simulink model "UScityblock2_Intersection"  (R2021b)
settings: Solver=ode23s  StartTime=0.0  StopTime=25  RelTol=1e-3
model workspace (MAT data in the model file):
  firstWarning = 1
  originalScenarioChecksum = '44EB4239245A86A3DA7E3FEB76A9F5A7'
values from neighbouring files (symbols this model uses):
  curvature = (DX.*D2Y - DY.*D2X) ./(DX.^2+DY.^2).^(3/2)    [setUpModel_UScityblock2.m]
  direction = ones(length(gradbp),1)    [setUpModel_UScityblock2.m]
  gradbp = linspace(0,totalDistance,50)    [setUpModel_UScityblock2.m]
  psi_o = thetaRefab(1)*(pi/180)    [setUpModel_UScityblock2.m]
  speed_actor1_gdps = smooth(speedgradbpactor1,speedactor1le)    [velocity_profiles.m]
  speed_actor2_gdps = smooth(speedgradbpactor2,speedactor2le)    [velocity_profiles.m]
  speed_actor3_gdps = smooth(speedgradbpactor3,speedactor3le)    [velocity_profiles.m]
  speed_actor4_gdps = smooth(speedgradbpactor4,speedactor4le)    [velocity_profiles.m]
  speed_ego_gdps = smooth(speedgradbpego,speedegole)    [velocity_profiles.m]
  thetaRefab = zeros(length(gradbp),1)    [setUpModel_UScityblock2.m]
  x_gdps = smooth(gradbp,xwaypoints)    [setUpModel_UScityblock2.m]
  X_o = x_ego_i(1)    [setUpModel_UScityblock2.m]
  y_gdps = smooth(gradbp,ywaypoints)    [setUpModel_UScityblock2.m]
  Y_o = y_ego_i(1)    [setUpModel_UScityblock2.m]
undefined symbols (not defined in the file or in its folder): distancecovered, gradbpA1, gradbpA2, gradbpA3, gradbpA4, gradbpego, magnitude, n, q11, v2xCA
libraries: drivingscenarioandsensors x7, sim3dautolib x5, vehdynlibtirecommon x4, autolibutils x4, aerolibconvert2 x2, simulink_extras x2, drivingvehiclecontroller x2, sim3dlib x1, vehdynlibtire x1, simulink x1, autolibshared x1
(part 2 of 2)

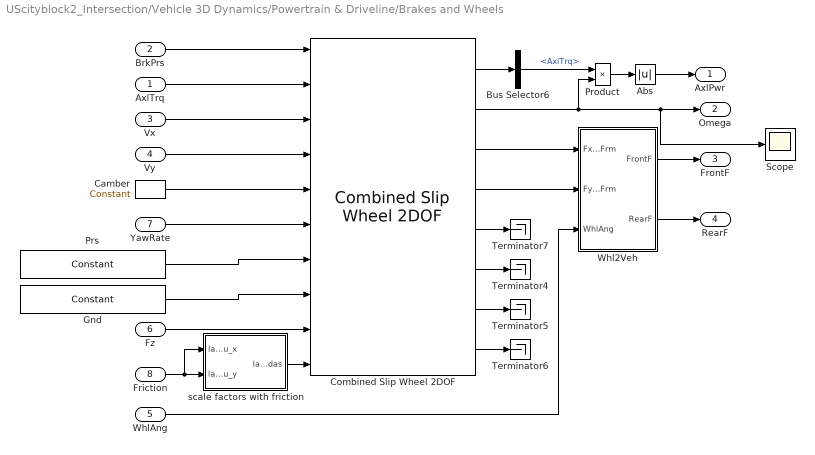
== system UScityblock2_Intersection/Vehicle 3D Dynamics/Powertrain & Driveline/Brakes and Wheels ==
  AxlTrq : Inport
  BrkPrs : Inport  Port=2
  Vx : Inport  Port=3
  Vy : Inport  Port=4
  WhlAng : Inport  Port=5
  Fz : Inport  Port=6  PortDimensions=4
  YawRate : Inport  Port=7
  Friction : Inport  Port=8
  Abs : Abs
  Bus Selector6 : BusSelector  OutputSignals=AxlTrq
  Camber : vehdynlibtirecommon/Constant  const=0  numWheels=4
      settings: SourceProductBaseCode=VE
  Combined Slip Wheel 2DOF : vehdynlibtire/Combined Slip Wheel 2DOF  tireType=External file  BrakeType=Disc  plySteer=off  turnslip=off  mu_static=.3  mu_kinetic=.2  disk_abore=.05  Rm=.177  num_pads=2  drum_abore=0.0508  drum_a=0.123  drum_c=0.212  drum_r=0.15  drum_theta1=0  drum_theta2=126  brake_p_bpt=[1 11.4736842105263 21.9473684210526 32.4210526315789 42.8947368421053 53.3684210526316 63.8421052631579 74.3157894736842 84.7894736842105 95.2631578947368 105.736842105263 116.210526315789 126.684210526316 137.157894736842 147.631578947368 158.105263157895 168.578947368421 179.052631578947 189.526315789474 200]  brake_n_bpt=[0 52.6315789473684 105.263157894737 157.894736842105 210.526315789474 263.157894736842 315.789473684211 368.421052631579 421.052631578947 473.684210526316 526.315789473684 578.947368421053 631.578947368421 684.210526315789 736.842105263158 789.473684210526 842.105263157895 894.736842105263 947.368421052632 1000]  f_brake_t=[43.4900602404453 42.5056030554862 41.5350898940194 40.5780454442085 39.6340111501808 38.7025443887544 37.7832176914519 36.8756180088306 35.9793460143796 35.0940154454303 34.2192524787115 33.3546951383474 32.4999927342521 31.6548053290159 30.8188032315107 29.991666515561 29.1730845621415 28.362755623661 27.5603864089927 26.765691687993;498.991217495636 487.695866636631 476.560505099801 465.579679307235 454.748127933653 444.060772460445 433.51270824929 423.099196101319 412.81565427025 402.657650900201 392.620896861006 382.701238955775 372.894653477208 363.197240090814 353.605216024701 344.114910546964 334.722759712992 325.425301366216 316.219170376863 307.10109410434;954.492374750826 932.886130217776 911.585920305583 890.581313170261 869.862244717126 849.419000532136 829.242198807128 809.322774193808 789.651962526121 770.221286354971 751.0225412433 732.047782773203 713.289314220164 694.739674852612 676.391628817892 658.238154578366 640.272434863842 622.48784710877 604.877954344734 587.436496520688;1409.99353200602 1378.07639379892 1346.61133551136 1315.58294703329 1284.9763615006 1254.77722860383 1224.97168936497 1195.5463522863 1166.48827078199 1137.78492180974 1109.42418562559 1081.39432659063 1053.68397496312 1026.28210961441 999.178041611083 972.361398609768 945.822110014692 919.550392851325 893.536738312604 867.771898937035;1865.49468926121 1823.26665738007 1781.63675071715 1740.58458089631 1700.09047828407 1660.13545667552 1620.7011799228 1581.76993037878 1543.32457903786 1505.34855726451 1467.82583000789 1430.74087040806 1394.07863570608 1357.82454437621 1321.96445440427 1286.48464264117 1251.37178516554 1216.61293859388 1182.19552228048 1148.10730135338;2320.9958465164 2268.45692096121 2216.66216592293 2165.58621475934 2115.20459506754 2065.49368474721 2016.43067048064 1967.99350847127 1920.16088729373 1872.91219271928 1826.22747439018 1780.08741422549 1734.47329644903 1689.36697913801 1644.75086719747 1600.60788667257 1556.92146031639 1513.67548433643 1470.85430624835 1428.44270376973;2776.49700377159 2713.64718454235 2651.68758112871 2590.58784862237 2530.31871185102 2470.8519128189 2412.16016103848 2354.21708656376 2296.9971955496 2240.47582817405 2184.62911877248 2129.43395804292 2074.86795719199 2020.9094138998 1967.53727999066 1914.73113070398 1862.47113546724 1810.73803007899 1759.51309021622 1708.77810618608;3231.99816102678 3158.8374481235 3086.71299633449 3015.58948248539 2945.43282863449 2876.21014089059 2807.88965159632 2740.44066465625 2673.83350380547 2608.03946362882 2543.03076315477 2478.78050186034 2415.26261793494 2352.4518486616 2290.32369278385 2228.85437473538 2168.02081061809 2107.80057582154 2048.17187418409 1989.11350860242;3687.49931828197 3604.02771170464 3521.73841154027 3440.59111634842 3360.54694541796 3281.56836896228 3203.61914215416 3126.66424274874 3050.66981206134 2975.60309908359 2901.43240753707 2828.12704567777 2755.6572786779 2683.9942834234 2613.11010557704 2542.97761876678 2473.57048576894 2404.8631215641 2336.83065815196 2269.44891101877;4143.00047553716 4049.21797528579 3956.76382674606 3865.59275021144 3775.66106220143 3686.92659703397 3599.34863271199 3512.88782084123 3427.50612031721 3343.16673453836 3259.83405191936 3177.4735894952 3096.05193942085 3015.5367181852 2935.89651837023 2857.10086279818 2779.12016091979 2701.92566730665 2625.48944211983 2549.78431343512;4598.50163279235 4494.40823886693 4391.78924195184 4290.59438407447 4190.77517898491 4092.28482510566 3995.07812326983 3899.11139893372 3804.34242857308 3710.73036999313 3618.23569630166 3526.82013331263 3436.44660016381 3347.079152947 3258.68293116342 3171.22410682959 3084.66983607064 2998.98821304921 2914.1482260877 2830.11971585147;5054.00279004754 4939.59850244808 4826.81465715762 4715.59601793749 4605.88929576838 4497.64305317735 4390.80761382767 4285.3349770262 4181.17873682896 4078.2940054479 3976.63734068395 3876.16667713006 3776.84126090677 3678.62158770879 3581.46934395661 3485.34735086099 ...(+2764 chars)]  tireParamSet=vdynPassCar.mat  PRESMAX=1003118  PRESMIN=9982  FZMAX=10000  FZMIN=100  VXLOW=.01  KPUMAX=1  KPUMIN=-1  ALPMAX=pi/2  ALPMIN=-pi/2  CAMMAX=0.173142086627737  CAMMIN=-0.173348165334087  LONGVL=16.7  FxRelFreqLwrLim=200*pi  FyRelFreqLwrLim=200*pi  MyRelFreqLwrLim=100*pi  omegao=10/.309  br=1e-3  UNLOADED_RADIUS=0.309  NOMPRES=224006  FNOMIN=4025  WIDTH=0.209  RIM_RADIUS=.19  MASS=9.465  IYY=0.7406  GRAVITY=-9.81  zo=0  zdoto=0  BREFF=8.25094594147963  DREFF=0.260468730454265  FREFF=0.0735298544471851  Q_RE0=1.00866439868088  Q_V1=0.000760413786224011  Q_V2=0.0463384792019201  Q_FZ1=0  Q_FZ2=15.6870832810226  Q_FZ3=0  Q_FCX=0.138643970247602  Q_FCY=0.10843499565426  Q_FCY2=-0.465763352339538  PFZ1=0.69958166705601  VERTICAL_STIFFNESS=207885.061134007  VERTICAL_DAMPING=494.649255786991  BOTTOM_OFFST=.01  BOTTOM_STIFF=2e6  LONGITUDINAL_STIFFNESS=388714.175879854  LATERAL_STIFFNESS=157087.404633332  PCFX1=0.18539229191199  PCFX2=0  PCFX3=0  PCFY1=0.163183345037677  PCFY2=0  PCFY3=0.249094918231954  Q_RA1=0.675942571700787  Q_RA2=0.73800463546164  Q_RB1=1.04487486456705  Q_RB2=-1.191763806629  PCX1=1.58523057950359  PDX1=1.0239116238178  PDX2=-0.0842405110022724  PDX3=0  PEX1=0.110312777158455  PEX2=0.313468516038146  PEX3=0  PEX4=0.0016060905760045  PKX1=21.3872544684023  PKX2=14.0006541873175  PKX3=-0.405326109653452  PHX1=0.000212599305364818  PHX2=0.00115950515263055  PVX1=1.59236164471432e-05  PVX2=0.000104321112127671  PPX1=-0.349461321276586  PPX2=0.387840040616429  PPX3=-0.0969947336569324  PPX4=0.0632271859795801  RBX1=12.7633329850276  RBX2=9.5787123658471  RBX3=0  RCX1=1.02796280922059  REX1=-0.45202516851367  REX2=-0.47304886171176  RHX1=0.000233272373115809  QSX1=-0.00788307788961443  QSX2=0.954629515459396  QSX3=0.0155855777667025  QSX4=0.125904607142414  QSX5=1.01110069703963  QSX6=20.1938577118433  QSX7=0.310818120717083  QSX8=-0.0430823751139655  QSX9=0.636494404888216  QSX10=0.142438060591663  QSX11=0.346766530036373  QSX12=0  QSX13=0  QSX14=0  PPMX1=0  PCY1=1.34299950037631  PDY1=0.878267729082195  PDY2=-0.0644597923147385  PDY3=0  PEY1=-0.809776534470972  PEY2=-0.600180598867198  PEY3=0.0991732552633487  PEY4=-6.5577974035573  PEY5=0  PKY1=-15.5714726518315  PKY2=1.73126522291751  PKY3=0.365349873517229  PKY4=1.98176755955416  PKY5=0  PKY6=-0.884005199550313  PKY7=-0.237259727611847  PHY1=-0.00183370557235628  PHY2=0.00346401302716671  PVY1=-0.00675427560163264  PVY2=0.036379218103843  PVY3=-0.163543984089166  PVY4=-0.491003349625726  PPY1=-0.62059646553185  PPY2=-0.0647824842338686  PPY3=-0.164648843290686  PPY4=0.283193909060098  PPY5=0  RBY1=10.7588809173639  RBY2=7.70420065295029  RBY3=3.40283755070691e-06  RBY4=0  RCY1=1.06691874059059  REY1=0.308244924574305  REY2=7.48775032604508e-06  RHY1=0.0118479204960415  RHY2=7.63650177161071e-06  RVY1=0.0560024425050078  RVY2=7.48487127056197e-06  RVY3=0  RVY4=98.4047026517149  RVY5=2.02759273900054  RVY6=15.7623064923347  QSY1=0.00699077564863536  QSY2=0  QSY3=0.00153535478298811  QSY4=8.55710322455322e-05  QSY5=0  QSY6=0  QSY7=0.89443879773793  QSY8=-0.403227641260894  QBZ1=11.666656027484  QBZ2=-1.30355438574485  QBZ3=0  QBZ4=0.177918305399071  QBZ5=-0.162481135068033  QBZ6=0  QBZ9=30.1445534682089  QBZ10=0  QCZ1=1.29026978207574  QDZ1=0.0886972644991399  QDZ2=-0.0058634820161856  QDZ3=0.3805597481383  QDZ4=0  QDZ6=0.00160914918118959  QDZ7=-0.00211036330862154  QDZ8=-0.13921904912557  QDZ9=0.00816585550028243  QDZ10=0  QDZ11=0  QEZ1=-2.19802254534746  QEZ2=1.01850535789165  QEZ3=0  QEZ4=0.278379679112054  QEZ5=-0.548414722765386  QHZ1=0.00148361198869669  QHZ2=0.00202017567585904  QHZ3=0.240316641332066  QHZ4=-0.210114035738085  PPZ1=-0.443927982388615  PPZ2=0  SSZ1=0.00914999585397887  SSZ2=0.0389830656052735  SSZ3=0  SSZ4=0  PDXP1=0.396718274678791  PDXP2=0  PDXP3=0  PKYP1=1.00587060633573  PDYP1=0.40483048923438  PDYP2=0  PDYP3=0  PDYP4=0  PHYP1=0.992731942067188  PHYP2=0.150352945499914  PHYP3=0  PHYP4=-3.98988682633674  PECP1=0.502379254513503  PECP2=0  QDTP1=10.0178654287947  QCRP1=0.200627747200702  QCRP2=0.0995735881599772  QBRP1=0.0997107127960717  QDRP1=1.01432910167423  QDRP2=0  aMode=2
      settings: SourceProductBaseCode=VE
  Gnd : vehdynlibtirecommon/Constant  const=0  numWheels=4
      settings: SourceProductBaseCode=VE
  Product : Product
  Prs : vehdynlibtirecommon/Constant  const=2.4e5  numWheels=4
      settings: SourceProductBaseCode=VE
  Scope : Scope
  Terminator{4..7} (4 alike) : Terminator
  Whl2Veh : Subsystem
  scale factors with friction : Subsystem  mask{numWheels=4}
      mask prompts: numWheels "Number of wheels"
  AxlPwr : Outport
  Omega : Outport  Port=2
  FrontF : Outport  Port=3
  RearF : Outport  Port=4
  wires:
  scale factors with friction/1(lambdas) -> Combined Slip Wheel 2DOF/10
  Whl2Veh/2(RearF) -> RearF/1
  Whl2Veh/1(FrontF) -> FrontF/1
  Bus Selector6/1 -> Product/1  "<AxlTrq>"
  Abs/1 -> AxlPwr/1
  Combined Slip Wheel 2DOF/4 -> Whl2Veh/2(FyWhlFrm)
  Friction/1 -> scale factors with friction/2(lamda_mu_y), scale factors with friction/1(lamda_mu_x)
  Prs/1 -> Combined Slip Wheel 2DOF/7
  Combined Slip Wheel 2DOF/8 -> Terminator6/1
  Combined Slip Wheel 2DOF/5 -> Terminator7/1
  YawRate/1 -> Combined Slip Wheel 2DOF/6
  Combined Slip Wheel 2DOF/3 -> Whl2Veh/1(FxWhlFrm)
  AxlTrq/1 -> Combined Slip Wheel 2DOF/2
  Vy/1 -> Combined Slip Wheel 2DOF/4
  Vx/1 -> Combined Slip Wheel 2DOF/3
  Fz/1 -> Combined Slip Wheel 2DOF/9
  WhlAng/1 -> Whl2Veh/3(WhlAng)
  Product/1 -> Abs/1
  BrkPrs/1 -> Combined Slip Wheel 2DOF/1
  Combined Slip Wheel 2DOF/6 -> Terminator4/1
  Camber/1 -> Combined Slip Wheel 2DOF/5
  Combined Slip Wheel 2DOF/7 -> Terminator5/1
  Combined Slip Wheel 2DOF/2 -> Product/2, Scope/1, Omega/1
  Combined Slip Wheel 2DOF/1 -> Bus Selector6/1
  Gnd/1 -> Combined Slip Wheel 2DOF/8

== system UScityblock2_Intersection/Vehicle 3D Dynamics/Powertrain & Driveline/Driveline ==
  TPowertrain : Inport  PortDimensions=1
  Gear : Inport  Port=2
  AWD : Subsystem  VariantControl=2
  FWD : Subsystem  VariantControl=1
  RWD : Subsystem  VariantControl=0
  TAxles : Outport  PortDimensions=4  VectorParamsAs1DForOutWhenUnconnected=off

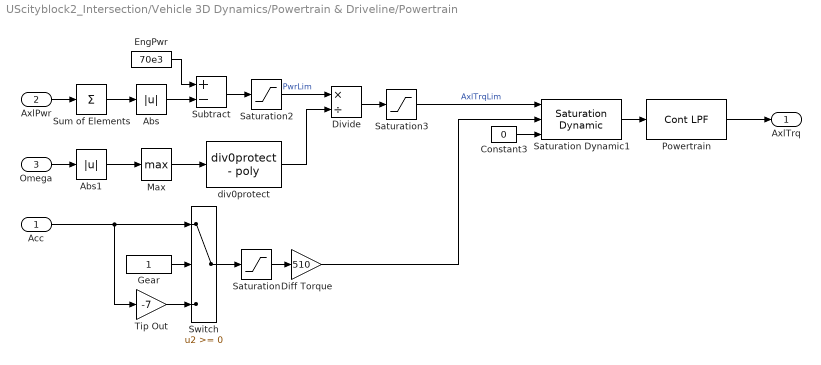
== system UScityblock2_Intersection/Vehicle 3D Dynamics/Powertrain & Driveline/Powertrain ==
  Acc : Inport
  AxlPwr : Inport  Port=2  PortDimensions=4
  Omega : Inport  Port=3  PortDimensions=4
  Abs : Abs  ZeroCross=off
  Abs1 : Abs  ZeroCross=off
  Constant3 : Constant  Value=0
  Diff Torque : Gain  Gain=510
  Divide : Product  Inputs=*/
  EngPwr : Constant  Value=70e3
  Gear : Constant  SampleTime=-1
  Max : MinMax  Function=max  ZeroCross=off
  Powertrain : autolibutils/Cont LPF  wc=4*pi*2  aMode=2
      settings: SourceProductBaseCode=PW,DR,MT,UV,VE
  Saturation : Saturate  UpperLimit=inf  LowerLimit=0  ZeroCross=off
  Saturation Dynamic1 : simulink/Discontinuities/Saturation Dynamic  OutMin=[]  OutMax=[]  OutDataTypeStr=Inherit: Same as second input  OutDataType=fixdt(1, 16)  OutScaling=2^-10  DoSatur=off
  Saturation2 : Saturate  UpperLimit=inf  LowerLimit=100  ZeroCross=off
  Saturation3 : Saturate  UpperLimit=1000  LowerLimit=0  ZeroCross=off
  Subtract : Sum  Inputs=+-
  Sum of Elements : Sum  Inputs=+
  Switch : Switch  ZeroCross=off
  Tip Out : Gain  Gain=-7
  div0protect : autolibutils/div0protect - poly  thresh=1  ZeroCross1=off  aMode=2
      settings: SourceProductBaseCode=PW,DR,MT,UV,VE
  AxlTrq : Outport  VectorParamsAs1DForOutWhenUnconnected=off
  wires:
  Abs1/1 -> Max/1
  Max/1 -> div0protect/1
  Saturation3/1 -> Saturation Dynamic1/1  "AxlTrqLim"
  AxlPwr/1 -> Sum of Elements/1
  EngPwr/1 -> Subtract/1
  Saturation2/1 -> Divide/1  "PwrLim"
  Subtract/1 -> Saturation2/1
  Omega/1 -> Abs1/1
  div0protect/1 -> Divide/2
  Divide/1 -> Saturation3/1
  Abs/1 -> Subtract/2
  Sum of Elements/1 -> Abs/1
  Constant3/1 -> Saturation Dynamic1/3
  Tip Out/1 -> Switch/3
  Saturation Dynamic1/1 -> Powertrain/1
  Gear/1 -> Switch/2
  Diff Torque/1 -> Saturation Dynamic1/2
  Saturation/1 -> Diff Torque/1
  Acc/1 -> Switch/1, Tip Out/1
  Switch/1 -> Saturation/1
  Powertrain/1 -> AxlTrq/1

== system UScityblock2_Intersection/Vehicle 3D Dynamics/Powertrain & Driveline/Vehicle to Tire ==
  VehFdbk : Inport
  WhlAng : Inport  Port=2
  Bus Selector : BusSelector  OutputSignals=BdyFrm.FrntAxl.Lft.Vel.xdot,BdyFrm.FrntAxl.Rght.Vel.xdot,BdyFrm.RearAxl.Lft.Vel.xdot,BdyFrm.RearAxl.Rght.Vel.xdot,BdyFrm.FrntAxl.Lft.Vel.ydot,BdyFrm.FrntAxl.Rght.Vel.ydot,BdyFrm.RearAxl.Lft.Vel.ydot,BdyFrm.RearAxl.Rght.Vel.ydot
  Mux : Mux
  Mux2 : Mux
  Veh2Whl : Subsystem
  WhlVelx : Outport
  WhlVel : Outport  Port=2
  wires:
  WhlAng/1 -> Veh2Whl/3(WhlAng)
  Veh2Whl/2(VyWhlFrm) -> WhlVel/1
  Veh2Whl/1(VxWhlFrm) -> WhlVelx/1
  Mux2/1 -> Veh2Whl/2(Vy)
  Mux/1 -> Veh2Whl/1(Vx)
  VehFdbk/1 -> Bus Selector/1
  Bus Selector/1 -> Mux/1  "<xdot>"
  Bus Selector/7 -> Mux2/3  "<ydot>"
  Bus Selector/8 -> Mux2/4  "<ydot>"
  Bus Selector/6 -> Mux2/2  "<ydot>"
  Bus Selector/4 -> Mux/4  "<xdot>"
  Bus Selector/2 -> Mux/2  "<xdot>"
  Bus Selector/3 -> Mux/3  "<xdot>"
  Bus Selector/5 -> Mux2/1  "<ydot>"

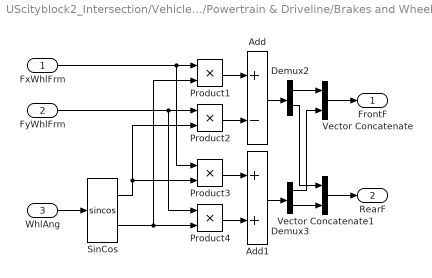
== system UScityblock2_Intersection/Vehicle 3D Dynamics/Powertrain & Driveline/Brakes and Wheels/Whl2Veh ==
  FxWhlFrm : Inport  PortDimensions=4
  FyWhlFrm : Inport  Port=2  PortDimensions=4
  WhlAng : Inport  Port=3
  Add : Sum  Inputs=+-
  Add1 : Sum
  Demux2 : Demux  Outputs=[2 2]
  Demux3 : Demux  Outputs=[2 2]
  Product{1..4} (4 alike) : Product
  SinCos : Trigonometry  Operator=sincos
  Vector Concatenate : Concatenate  Mode=Multidimensional array  ConcatenateDimension=2
  Vector Concatenate1 : Concatenate  Mode=Multidimensional array  ConcatenateDimension=2
  FrontF : Outport
  RearF : Outport  Port=2
  wires:
  Vector Concatenate/1 -> FrontF/1
  Demux3/1 -> Vector Concatenate/2
  Demux2/1 -> Vector Concatenate/1
  Demux2/2 -> Vector Concatenate1/1
  Demux3/2 -> Vector Concatenate1/2
  Vector Concatenate1/1 -> RearF/1
  Product4/1 -> Add1/2
  Add/1 -> Demux2/1
  Product2/1 -> Add/2
  SinCos/1 -> Product2/2, Product3/2
  Product1/1 -> Add/1
  SinCos/2 -> Product4/2, Product1/2
  FyWhlFrm/1 -> Product4/1, Product2/1
  Add1/1 -> Demux3/1
  FxWhlFrm/1 -> Product3/1, Product1/1
  Product3/1 -> Add1/1
  WhlAng/1 -> SinCos/1

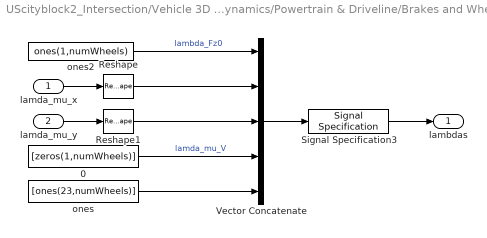
== system UScityblock2_Intersection/Vehicle 3D Dynamics/Powertrain & Driveline/Brakes and Wheels/scale factors with friction ==
  lamda_mu_x : Inport
  lamda_mu_y : Inport  Port=2
  0 : Constant  Value=[zeros(1,numWheels)]  VectorParams1D=off
  Reshape : Reshape  OutputDimensionality=Row vector (2-D)  OutputDimensions=[1,numWheels]
  Reshape1 : Reshape  OutputDimensionality=Row vector (2-D)  OutputDimensions=[1,numWheels]
  Signal Specification3 : SignalSpecification  Unit=1
  Vector Concatenate : Concatenate  NumInputs=5  Mode=Multidimensional array
  ones : Constant  Value=[ones(23,numWheels)]  VectorParams1D=off
  ones2 : Constant  Value=ones(1,numWheels)  VectorParams1D=off
  lambdas : Outport  Unit=1  VectorParamsAs1DForOutWhenUnconnected=off
  wires:
  Signal Specification3/1 -> lambdas/1
  Reshape/1 -> Vector Concatenate/2
  Reshape1/1 -> Vector Concatenate/3
  0/1 -> Vector Concatenate/4  "lamda_mu_V"
  ones/1 -> Vector Concatenate/5
  Vector Concatenate/1 -> Signal Specification3/1
  ones2/1 -> Vector Concatenate/1  "lambda_Fz0"
  lamda_mu_x/1 -> Reshape/1
  lamda_mu_y/1 -> Reshape1/1

== system UScityblock2_Intersection/Vehicle 3D Dynamics/Powertrain & Driveline/Driveline/AWD ==
  TPowertrain : Inport
  Gear : Inport  Port=2
  AWD : Gain  Gain=[1;1;1;1]./2
  Add : Sum
  Constant : Constant
  Constant1 : Constant  Value=zeros(4,1)
  Multiport Switch : MultiPortSwitch  DataPortOrder=Zero-based contiguous  zeroidx=on
  Unary Minus : UnaryMinus
  TAxles : Outport  VectorParamsAs1DForOutWhenUnconnected=off
  wires:
  Unary Minus/1 -> Multiport Switch/2
  Gear/1 -> Add/1
  Constant/1 -> Add/2
  AWD/1 -> Multiport Switch/4, Unary Minus/1
  Constant1/1 -> Multiport Switch/3
  Add/1 -> Multiport Switch/1
  Multiport Switch/1 -> TAxles/1
  TPowertrain/1 -> AWD/1

== system UScityblock2_Intersection/Vehicle 3D Dynamics/Powertrain & Driveline/Driveline/FWD ==
  TPowertrain : Inport
  Gear : Inport  Port=2
  Add : Sum
  Constant : Constant
  Constant1 : Constant  Value=zeros(4,1)
  FWD : Gain  Gain=[1;1;0;0]
  Multiport Switch : MultiPortSwitch  DataPortOrder=Zero-based contiguous  zeroidx=on
  Unary Minus : UnaryMinus
  TAxles : Outport  VectorParamsAs1DForOutWhenUnconnected=off
  wires:
  Unary Minus/1 -> Multiport Switch/2
  Gear/1 -> Add/1
  Constant/1 -> Add/2
  FWD/1 -> Multiport Switch/4, Unary Minus/1
  Constant1/1 -> Multiport Switch/3
  Add/1 -> Multiport Switch/1
  Multiport Switch/1 -> TAxles/1
  TPowertrain/1 -> FWD/1

== system UScityblock2_Intersection/Vehicle 3D Dynamics/Powertrain & Driveline/Driveline/RWD ==
  TPowertrain : Inport
  Gear : Inport  Port=2
  Add : Sum
  Constant : Constant
  Constant1 : Constant  Value=zeros(4,1)
  Multiport Switch : MultiPortSwitch  DataPortOrder=Zero-based contiguous  zeroidx=on
  RWD : Gain  Gain=[0;0;1;1]
  Unary Minus : UnaryMinus
  TAxles : Outport  VectorParamsAs1DForOutWhenUnconnected=off
  wires:
  Constant1/1 -> Multiport Switch/3
  Add/1 -> Multiport Switch/1
  Constant/1 -> Add/2
  Gear/1 -> Add/1
  Multiport Switch/1 -> TAxles/1
  Unary Minus/1 -> Multiport Switch/2
  TPowertrain/1 -> RWD/1
  RWD/1 -> Multiport Switch/4, Unary Minus/1

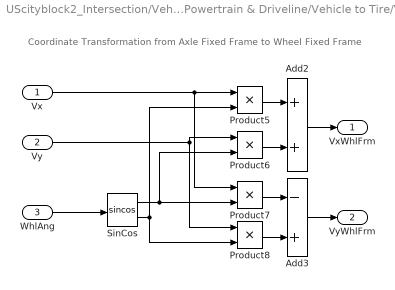
== system UScityblock2_Intersection/Vehicle 3D Dynamics/Powertrain & Driveline/Vehicle to Tire/Veh2Whl ==
  note: Coordinate Transformation from Axle Fixed Frame to Wheel Fixed Frame
  Vx : Inport
  Vy : Inport  Port=2
  WhlAng : Inport  Port=3
  Add2 : Sum
  Add3 : Sum  Inputs=-+
  Product{5..8} (4 alike) : Product
  SinCos : Trigonometry  Operator=sincos
  VxWhlFrm : Outport
  VyWhlFrm : Outport  Port=2
  wires:
  Add2/1 -> VxWhlFrm/1
  Add3/1 -> VyWhlFrm/1
  Product7/1 -> Add3/1
  Vy/1 -> Product8/1, Product6/1
  SinCos/2 -> Product8/2, Product5/2
  SinCos/1 -> Product7/2, Product6/2
  Product5/1 -> Add2/1
  Product6/1 -> Add2/2
  Product8/1 -> Add3/2
  Vx/1 -> Product5/1, Product7/1
  WhlAng/1 -> SinCos/1

== matlab function UScityblock2_Intersection/MATLAB Function ==
  data: VX_EGO output; vxi input; vxj input; vxk input; vxl input
function VX_EGO = Collision_Avoidance(vxi,vxj,vxk,vxl)


%%%%%%%%%%%%%%%%%%%%%%%%%%%%%%%%%%%%%%%%%%%%%%%%%%%%%%%%%%%%%%%%%%%%%%%%%
%%%%%%%%%%%%%%%%%%%%%%%%%%%%%%%%%%%%%%%%%%%%%%%%%%%%%%%%%%%%%%%%%%%%%%%%%
%%%%%%%%%%%%%%%%%%%%%%%%%%%%%%%%%%%%%%%%%%%%%%%%%%%%%%%%%%%%%%%%%%%%%%%%

%let V1 is ego vehicle,  V1=[lonituginal position,lateral position,
% longitudinal velocity,lateral velocity,heading, turn indication, 
% lane indication, forward length of vehicle from cg,
%input = time
%CA = zeros(t)
%for CA = 1:t
    
     

% rear length from cg, width of vehicle, alocated time slot] 
% therefore V1=[x,y,vx,vy,sai,I,L,lf,lr,w,f1]
lf=4 % vehicle front length from cg 
lr=4 % vehicle rear length from cg
S1=[1,-2] % lane i starting point
S2=[2,1]% lane j starting point
S3=[-1,2]% lane k starting point
S4=[-2,-1] % lane l starting point
S=[S1,S2,S3,S4] % start cordinate points for each lane i,j,k,l respectively 
f1=1 % time alocation for ego in lane i
f2=1 % time alocation for actor in lane j
f3=1 % time alocation for actor in lane k
f4=1 % time alocation for actor in lane l
f11=1 % time alocation for actor in lane i second vehicle
f=[f11,f1,f2,f3,f4]
ilR=10 % left path radius in fts = 33 is 10 meters
irR=5 % right path radius in fts= 16 is 5 meters
sR=5 % straight path distance
il=1 % left turn indication in values
ir=2 % right turn indication in values
is=3 % straight pass indication in values

P1=3 % straight pass phase of traffic signal
P2=1 % left turn phase of traffic signal
P3=2 % right turn phase for traffic signal
P=[P1,P2,P3]% phase of the traffic signal
pi=P2 % phase for I lane
pj=P1 % phase for j lane
pk=P3 % phase for k lane
pl=P2 % phase for l lane
I=[il,ir,is] % turn indication
% vehicle parameters with values 
lf=1.3 % in meters 4ft = 1.3meters front length from cg
lr=1.3 % rear length from cg
w=1.3 % width of vehicle
% V1=[1,-2,10,0,90,il,S1,lf,lr,w,f1];
% V2=[2,1,10,0,180,is,S2,lf,lr,w,f2];
% V3=[-1,2,10,0,270,ir,S3,lf,lr,w,f3];
% V4=[-2,-1,10,0,0,il,S4,lf,lr,w,f4];
%turn indication
li=il % left
lj=is % straight
lk=ir % right
ll=il % left

prob1 = optimproblem('ObjectiveSense','minimize');
prob2 = optimproblem('ObjectiveSense','minimize');
prob3 = optimproblem('ObjectiveSense','minimize');
prob4 = optimproblem('ObjectiveSense','minimize');
vx = optimvar('vx',1,'LowerBound',1,'UpperBound',50,'Type','continuous');
show (vx)
%vx=15
e_i1=2^abs(li-pi)
e_j1=2^abs(lj-pj)
e_k1=2^abs(lk-pk)
e_l1=2^abs(ll-pl)
tawi=(lr+w/2)/vx
% vxi=speed_actor1_gdps(time)
% vxj=speed_actor2_gdps(time)
% vxk=speed_actor3_gdps(time)
% vxl=speed_actor4_gdps(time)


tawi_a=(lf+w/2)/vxi
tawj_a=(lf+w/2)/vxj
tawk_a=(lf+w/2)/vxk
tawl_a=(lf+w/2)/vxl
Ti_a= ((totalDistanceA4)/vxi)+tawi_a
Tj_a= (totalDistanceA1/vxj)+tawj_a
Tk_a= ((totalDistanceA2)/vxk)+tawk_a
Tl_a= (((totalDistanceA3)/2)/vxl)+tawl_a
Ti_e= ((totalDistanceego)/vx)+tawi

% zeta_i=abs((e_i1*(f1+Ti_e))-(e_i1*(f11+Ti_a))) 
% zeta_j=abs((e_j1*(f1+Ti_e))-(e_i1*(f2+Tj_a)))
% zeta_k=abs((e_k1*(f1+Ti_e))-(e_i1*(f3+Tk_a)))
% zeta_l=abs((e_l1*(f1+Ti_e))-(e_i1*(f4+Tl_a)))
%zeta1= zeta_i+zeta_j+zeta_k+zeta_l


%optimization problem









% prob = optimproblem('ObjectiveSense','maximize');
% vx(1) = optimvar('vx',1,'LowerBound',10,'UpperBound',30,'Type','continuous');
%prob.Objective = ((e_i1*(f1+(((ilR*pi)/2)/vx(1))+(lr+w/2)/vx(1)))-(e_i1*(f11+Ti_a)))+((e_j1*(f1+(((ilR*pi)/2)/vx(1))+(lr+w/2)/vx(1)))-(e_i1*(f2+Tj_a)))+((e_k1*(f1+(((ilR*pi)/2)/vx(1))+(lr+w/2)/vx(1)))-(e_i1*(f3+Tk_a)))+((e_l1*(f1+(((ilR*pi)/2)/vx(1))+(lr+w/2)/vx(1)))-(e_i1*(f4+Tl_a)));
%prob.Objective =zeta_i+zeta_j+zeta_k+zeta_l
% prob.Objective = abs((e_i1*(f1+(((ilR*pi)/2)/vx(1))+(lr+w/2)/vx(1)))-(e_i1*(f11+Ti_a)))+abs((e_j1*(f1+(((ilR*pi)/2)/vx(1))+(lr+w/2)/vx(1)))-(e_i1*(f2+Tj_a)))+abs((e_k1*(f1+(((ilR*pi)/2)/vx(1))+(lr+w/2)/vx(1)))-(e_i1*(f3+Tk_a)))+abs((e_l1*(f1+(((ilR*pi)/2)/vx(1))+(lr+w/2)/vx(1)))-(e_i1*(f4+Tl_a)));

zeta_i=(e_i1*(f1+(((totalDistanceego)/vx)))+ ((lr+w/2)/vx))-(e_i1*(f11+Ti_a))
zeta_j=(e_j1*(f1+(((totalDistanceego)/vx))+(lr+w/2)/vx))-(e_i1*(f2+Tj_a))
zeta_k=(e_k1*(f1+(((totalDistanceego)/vx))+(lr+w/2)/vx))-(e_i1*(f3+Tk_a))
zeta_l=((e_l1*(f1+(((totalDistanceego)/2)/vx))+(lr+w/2)/vx))-(e_i1*(f4+Tl_a))

%prob.Objective = (zeta_i + zeta_j + zeta_k + zeta_l)
prob1.Objective = sqrt((zeta_i)^2) 
prob2.Objective =  sqrt((zeta_j)^2) 
prob3.Objective = sqrt((zeta_k)^2)
prob4.Objective = sqrt((zeta_l)^2) 
cons1 = sqrt((zeta_i)^2) >= 0.07;
cons2 = sqrt((zeta_j)^2) >= 0.07;
cons3 = sqrt((zeta_k)^2) >= 0.07;
cons4 = sqrt((zeta_l)^2) >= 0.07;
cons5 = sqrt((zeta_i)^2) <= 5;
cons6 = sqrt((zeta_j)^2) <= 5;
cons7 = sqrt((zeta_k)^2) <= 5;
cons8 = sqrt((zeta_l)^2) <= 5;


% cons1 = -[(Ti_e+tawi)-(Ti_a+tawi_a)] >= 1;
%  cons2 =  (e_j1*(f1+(((ilR*pi)/2)/vx)+(lr+w/2)/vx(1)))-(e_i1*(f2+Tj_a)) >= 0.3;
%  cons3 =  ((e_k1*(f1+(((ilR*pi)/2)/vx)+(lr+w/2)/vx(1)))-(e_i1*(f3+Tk_a))) >= 0.3;
%  cons4 =  ((e_l1*(f1+(((ilR*pi)/2)/vx)+(lr+w/2)/vx(1)))-(e_i1*(f4+Tl_a))) >= 0.3;
% cons1 =  zeta_i >= 0.3;
% cons2 =  zeta_i <= 5;
% cons3 =  zeta_k >= 0.3;
% cons4 =   zeta_l >= 0.3;
% cons5 =  zeta_j >= 0.3;
% cons6 =  zeta_j <= 5;
% cons7 =  zeta_k <= 5;
% cons8 =   zeta_l <= 5;
% cons1 =  (e_i1*(f1+(((ilR*pi)/2)/vx)+(lr+w/2)/vx))-(e_i1*(f11+Ti_a)) >= 0.3;
% cons2 =  (e_j1*(f1+(((ilR*pi)/2)/vx)+(lr+w/2)/vx(1)))-(e_i1*(f2+Tj_a)) >= 0.3;
% cons3 =  ((e_k1*(f1+(((ilR*pi)/2)/vx)+(lr+w/2)/vx(1)))-(e_i1*(f3+Tk_a))) >= 0.3;
% cons4 =  ((e_l1*(f1+(((ilR*pi)/2)/vx)+(lr+w/2)/vx(1)))-(e_i1*(f4+Tl_a))) >= 0.3;
% cons5 =  ((e_i1*(f1+(((ilR*pi)/2)/vx)+(lr+w/2)/vx(1)))-(e_i1*(f11+Ti_a))) <= 10;
% cons6 =  ((e_j1*(f1+(((ilR*pi)/2)/vx)+(lr+w/2)/vx(1)))-(e_i1*(f2+Tj_a))) <= 10;
% cons7 =  ((e_k1*(f1+(((ilR*pi)/2)/vx)+(lr+w/2)/vx(1)))-(e_i1*(f3+Tk_a))) <= 10;
% cons8 = ((e_l1*(f1+(((ilR*pi)/2)/vx)+(lr+w/2)/vx(1)))-(e_i1*(f4+Tl_a))) <= 10;
%%%%%%%%%%%%%%%%%%%%%%%%%%%%%%%%
prob1.Constraints.cons1 = cons1;
prob1.Constraints.cons2 = cons2;
prob1.Constraints.cons3 = cons3;
prob1.Constraints.cons4 = cons4;
prob2.Constraints.cons1 = cons1;
prob2.Constraints.cons2 = cons2;
prob2.Constraints.cons3 = cons3;
prob2.Constraints.cons4 = cons4;
prob3.Constraints.cons1 = cons1;
prob3.Constraints.cons2 = cons2;
prob3.Constraints.cons3 = cons3;
prob3.Constraints.cons4 = cons4;
prob4.Constraints.cons1 = cons1;
prob4.Constraints.cons2 = cons2;
prob4.Constraints.cons3 = cons3;
prob4.Constraints.cons4 = cons4;
%%%%%%%%%%%%%%%%%%%%%%%%%%%%%%%%
prob1.Constraints.cons5 = cons5;
prob1.Constraints.cons6 = cons6;
prob1.Constraints.cons7 = cons7;
prob1.Constraints.cons8 = cons8;
prob2.Constraints.cons5 = cons5;
prob2.Constraints.cons6 = cons6;
prob2.Constraints.cons7 = cons7;
prob2.Constraints.cons8 = cons8;
prob3.Constraints.cons5 = cons5;
prob3.Constraints.cons6 = cons6;
prob3.Constraints.cons7 = cons7;
prob3.Constraints.cons8 = cons8;
prob4.Constraints.cons5 = cons5;
prob4.Constraints.cons6 = cons6;
prob4.Constraints.cons7 = cons7;
prob4.Constraints.cons8 = cons8;
%%%%%%%%%%%%%%%%%%%%%%%%%%%%%%%%
% prob.Constraints.cons5 = cons5;
% prob.Constraints.cons6 = cons6;
% prob.Constraints.cons7 = cons7;
% prob.Constraints.cons8 = cons8;
show(prob1)
show(prob2)
show(prob3)
show(prob4)
sol1 = solve(prob1,"Solver","surrogate")
sol2 = solve(prob2,"Solver","surrogate")

sol3 = solve(prob3,"Solver","surrogate")

sol4 = solve(prob4,"Solver","surrogate")

ans(1)=sol1.vx
ans(2)=sol2.vx
ans(3)=sol3.vx
ans(4)=sol4.vx
zeta_ii=((e_i1*(f1+((totalDistanceego)/ans(1))+(lr+w/2)/ans(1)))-(e_i1*(f11+Ti_a)))
zeta_jj=((e_j1*(f1+((totalDistanceego)/ans(2))+(lr+w/2)/ans(2)))-(e_i1*(f2+Tj_a)))
zeta_kk=((e_k1*(f1+((totalDistanceego)/ans(3))+(lr+w/2)/ans(3)))-(e_i1*(f3+Tk_a)))
zeta_ll=((e_l1*(f1+((totalDistanceego/2)/ans(4))+(lr+w/2)/ans(4)))-(e_i1*(f4+Tl_a)))
l123(CA)=zeta_ll
ii(CA)=zeta_ii
jj(CA)=zeta_jj
kk(CA)=zeta_kk



v2xCA=(ans(1)+ans(2)+ans(3)+ans(4))/4;


  %  end







%%%%%%%%%%%%%%%%%%%%%%%%%%%%%%%%%%%%%%%%%%%%%%%%%%%%%%%%%%%%%%%%%%%%%%%%%
%%%%%%%%%%%%%%%%%%%%%%%%%%%%%%%%%%%%%%%%%%%%%%%%%%%%%%%%%%%%%%%%%%%%%%%%%%

y = v2xCA;

== matlab function UScityblock2_Intersection/Subsystem2/MATLAB Function ==
  data: pos input; egoActor output Bus: BusActors1Actors; vel input; yaw input; yawRate input
function egoActor = packEgo(pos,vel,yaw,yawRate)
% Pack ego information into a single ego actor bus
%
% Imoprtant note:
% Output is a bus of type BusActorsActors. This is the same bus used by the
% Scenario Reader to output an individual actor. If you change the
% output bus name of Scenario Reader, change the output bus name here
% as well by clicking on 'Edit Data' in the menu above.

egoActor = struct(...
    'ActorID',1,...
    'Position', [pos(1) pos(2) 0], ...
    'Velocity', [vel(1) vel(2) 0], ...
    'Roll', 0, ...
    'Pitch', 0, ...
    'Yaw', yaw, ...
    'AngularVelocity', [0 0 yawRate]);
